simulink model "monitor_ceder_S0"  (R2025b)
settings: Solver=VariableStepDiscrete  StartTime=0.0  StopTime=100  RelTol=1e-3
values from neighbouring files (symbols this model uses):
  m = mean(ts.Data(idx))    [barrido_S0.m]
undefined symbols (not defined in the file or in its folder): n, periodGen
settings Model: Creator=ildio  LastModifiedBy=ildio

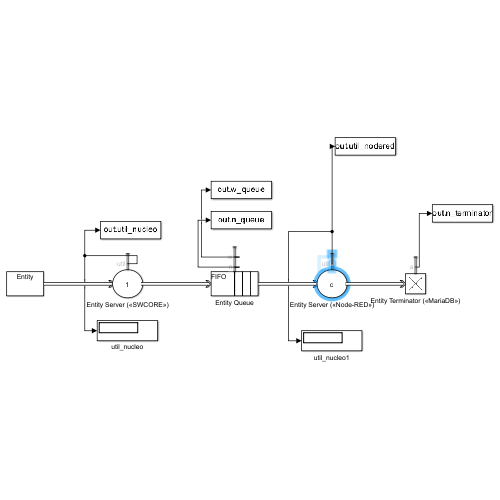
[thumbnail: Simulink's stored preview of the top-level diagram]
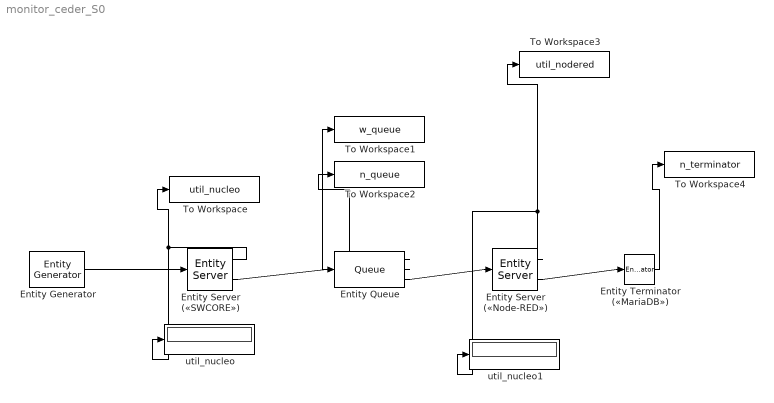
== system monitor_ceder_S0 ==
  Entity Generator : EntityGenerator  OutputPortMessageModes=m  Period=periodGen  EntityType=Structured  EntityTypeName=Entity
  Entity Queue : Queue  InputPortMessageModes=m  OutputPortMessageModes=n,n,m  Capacity=Inf  NumberEntitiesInBlock=on  AverageWait=on
      settings: OutputPortMap=o1,o2,o5
  Entity Server («Node-RED») : EntityServer  InputPortMessageModes=m  OutputPortMessageModes=n,m  Capacity=c  ServiceTimeValue=tResp  ServiceTimeAction=dt = -tResp .* log(rand(size(entitySys.id)));  Utilization=on
      settings: OutputPortMap=o5,o9
  Entity Server («SWCORE») : EntityServer  InputPortMessageModes=m  OutputPortMessageModes=n,m  Capacity=1  ServiceTimeValue=tNucleo  Utilization=on
      settings: OutputPortMap=o5,o9
  Entity Terminator («MariaDB») : EntityTerminator  InputPortMessageModes=m  NumberEntitiesArrived=on
      settings: OutputPortMap=o0
  To Workspace : ToWorkspace  VariableName=util_nucleo  SaveFormat=Timeseries  SampleTime=-1
      settings: Decimation=3
  To Workspace1 : ToWorkspace  VariableName=w_queue  SaveFormat=Timeseries  SampleTime=-1
      settings: Decimation=3
  To Workspace2 : ToWorkspace  VariableName=n_queue  SaveFormat=Timeseries  SampleTime=-1
      settings: Decimation=3
  To Workspace3 : ToWorkspace  VariableName=util_nodered  SaveFormat=Timeseries  SampleTime=-1
      settings: Decimation=3
  To Workspace4 : ToWorkspace  VariableName=n_terminator  SaveFormat=Timeseries  SampleTime=-1
      settings: Decimation=3
  util_nucleo : Display
  util_nucleo1 : Display
  wires:
  Entity Server («Node-RED»)/2 -> Entity Terminator («MariaDB»)/1
  Entity Queue/3 -> Entity Server («Node-RED»)/1
  Entity Generator/1 -> Entity Server («SWCORE»)/1
  Entity Server («SWCORE»)/2 -> Entity Queue/1
  Entity Server («SWCORE»)/1 -> util_nucleo/1, To Workspace/1
  Entity Server («Node-RED»)/1 -> To Workspace3/1, util_nucleo1/1
  Entity Queue/2 -> To Workspace1/1
  Entity Queue/1 -> To Workspace2/1
  Entity Terminator («MariaDB»)/1 -> To Workspace4/1
